simulink library "Vehicle_Axle1"  (R2026a)
settings: Solver=VariableStepAuto
undefined symbols (not defined in the file): Init, Trailer
libraries: Body_Utilities x1, Brakes_Axle1 x1, Chassis_Axle1 x1, Driveline_Axle1 x1, Power_Systems x1
Description:
  | Component of Simscape Vehicle Templates Library
  | 
  | Copyright 2018-2026 The MathWorks, Inc.
settings Model: Creator=smiller  LastModifiedBy=smiller

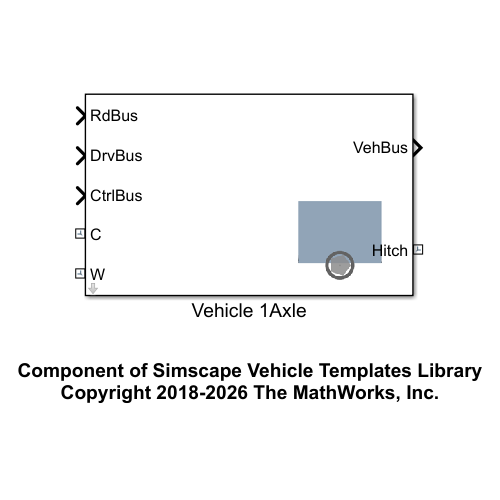
[thumbnail: Simulink's stored preview of the top-level diagram]
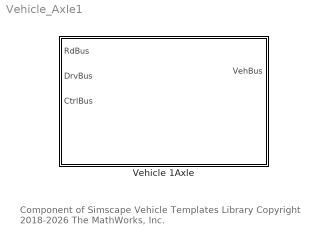
== system Vehicle_Axle1 ==
  note: Component of Simscape Vehicle Templates Library
      | Copyright 2018-2026 The MathWorks, Inc.
  Vehicle 1Axle : Subsystem  Tag=PublishSubsystem  VariantControl=NS_Con  mask(Vehicle with Single Axle){Vehicle=Trailer, Init=Init, veh_index=61}
      mask prompts: Vehicle "Vehicle Parameters"; Init "Initial Values"; veh_index "Vehicle Index (for tires)"
      mask help: Models vehicle with single axle with a multibody suspension. Initial Values data structure sets initial speed of wheels. Set tire index to ensures tire results can be saved independently from other vehicles in the model.
      mask Help: web('sm_car_doc_vehicle.html')
      mask TypeOptions veh_index: Chassis/veh_index
      mask DialogControl cont_sim Prompt: Config
      mask Display:
      | % Get image from BodyGeometry.class
      | % (active choice for Body Geometry subsystem)
      | temp_veh_bg_class = lower(get_param([gcb '/Chassis/Body/Body Geometry'],'LabelModeActiveChoice'));
      | 
      | imagestr = (['sm_car_vehicle_' temp_veh_bg_class '.png']);
      | if(~exist(imagestr))
      |     imagestr = ['sm_car_vehicle_axle1_default.png'];
      | end
      | 
      | image(imagestr);

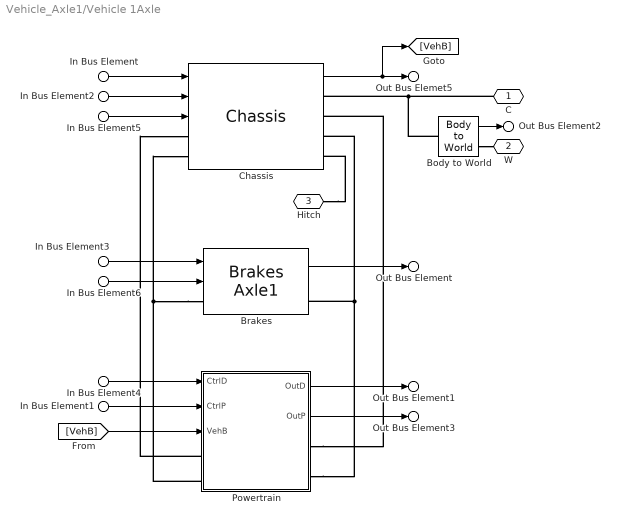
== system Vehicle_Axle1/Vehicle 1Axle ==
  In Bus Element2 : Inport  PortName=RdBus
  In Bus Element : Inport  Port=2  PortName=DrvBus
  In Bus Element3 : Inport  Port=2  PortName=DrvBus
  In Bus Element6 : Inport  Port=3  PortName=CtrlBus  Element=Brakes
  In Bus Element5 : Inport  Port=3  PortName=CtrlBus  Element=Chassis
  In Bus Element1 : Inport  Port=3  PortName=CtrlBus  Element=Power
  In Bus Element4 : Inport  Port=3  PortName=CtrlBus  Element=Driveline
  Body to World : Body_Utilities/Body to World  VariantControl=Choice  LabelModeActiveChoice=Free  popup_BodyToWorld=Free  SpecifyPosTarget=off
  Brakes : Brakes_Axle1/Brakes Axle1  VariantControl=Variant1  LabelModeActiveChoice=None  Brakes=Vehicle.Brakes  VariantLabel=Vehicle.Brakes.class.Value
      settings: AttributesFormatString=%<ActiveVariant>
  Chassis : Chassis_Axle1/Chassis  Tag=PublishSubsystem  VariantControl=Chassis  Chassis=Vehicle.Chassis  Init=Init  veh_index=veh_index
  Powertrain : Subsystem  mask{Powertrain=Vehicle.Powertrain}
      mask prompts: Powertrain "Powertrain Parameters"
  C : PMIOPort  Side=Left
  W : PMIOPort  Port=2  Side=Left
  Hitch : PMIOPort  Port=3  Side=Right
  Out Bus Elemet5 : Outport  VectorParamsAs1DForOutWhenUnconnected=off  PortName=VehBus  Element=Chassis
  Out Bus Element : Outport  VectorParamsAs1DForOutWhenUnconnected=off  PortName=VehBus  Element=Brakes
  Out Bus Element1 : Outport  VectorParamsAs1DForOutWhenUnconnected=off  PortName=VehBus  Element=Driveline
  Out Bus Element2 : Outport  VectorParamsAs1DForOutWhenUnconnected=off  PortName=VehBus  Element=World
  Out Bus Element3 : Outport  VectorParamsAs1DForOutWhenUnconnected=off  PortName=VehBus  Element=Power
  wires:
  [VehB] -> Powertrain/3(VehB)
  In Bus Element5/1 -> Chassis/3
  Brakes/1 -> Out Bus Element/1
  Chassis/1 -> [VehB], Out Bus Elemet5/1
  In Bus Element2/1 -> Chassis/2
  In Bus Element/1 -> Chassis/1
  In Bus Element6/1 -> Brakes/2
  Body to World/1 -> Out Bus Element2/1
  In Bus Element3/1 -> Brakes/1
  In Bus Element4/1 -> Powertrain/1(CtrlD)
  In Bus Element1/1 -> Powertrain/2(CtrlP)
  Powertrain/1(OutD) -> Out Bus Element1/1
  Powertrain/2(OutP) -> Out Bus Element3/1
  connections:
  Hitch/RConn1 -- Chassis/RConn4
  C/RConn1 -- Chassis/RConn1 -- Body to World/LConn1
  Body to World/RConn1 -- W/RConn1
  Brakes/RConn1 -- Chassis/RConn3 -- Powertrain/RConn2
  Brakes/LConn1 -- Chassis/LConn2 -- Powertrain/LConn2
  Powertrain/RConn1 -- Chassis/RConn2
  Powertrain/LConn1 -- Chassis/LConn1

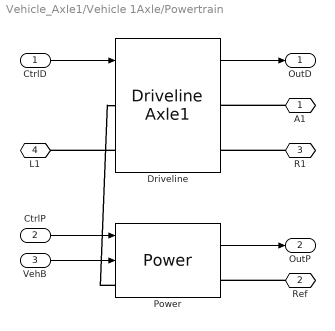
== system Vehicle_Axle1/Vehicle 1Axle/Powertrain ==
  CtrlD : Inport
  CtrlP : Inport  Port=2
  VehB : Inport  Port=3
  Driveline : Driveline_Axle1/Driveline Axle1  VariantControl=Shaft  LabelModeActiveChoice=None  Driveline=Vehicle.Powertrain.Driveline  VariantLabel=Vehicle.Powertrain.Driveline.class.Value
      settings: AttributesFormatString=%<ActiveVariant>
  Power : Power_Systems/Power  VariantControl=Variant1  LabelModeActiveChoice=None  Power=Powertrain.Power  VariantLabel=Powertrain.Power.class.Value
      settings: AttributesFormatString=%<ActiveVariant>
  A1 : PMIOPort  Side=Left
  Ref : PMIOPort  Port=2  Side=Right
  R1 : PMIOPort  Port=3  Side=Right
  L1 : PMIOPort  Port=4  Side=Left
  OutD : Outport  VectorParamsAs1DForOutWhenUnconnected=off
  OutP : Outport  Port=2  VectorParamsAs1DForOutWhenUnconnected=off
  wires:
  VehB/1 -> Power/2
  Driveline/1 -> OutD/1
  CtrlD/1 -> Driveline/1
  Power/1 -> OutP/1
  CtrlP/1 -> Power/1
  connections:
  Power/LConn1 -- Driveline/LConn1
  Ref/RConn1 -- Power/RConn1
  Driveline/LConn2 -- L1/RConn1
  A1/RConn1 -- Driveline/RConn1
  R1/RConn1 -- Driveline/RConn2
